simulink model "ep3_1"  (R2018a)
settings: Solver=VariableStepAuto  StartTime=0.0  StopTime=10.0  RelTol=1e-3
settings Model: Creator=zheny  LastModifiedBy=zheny

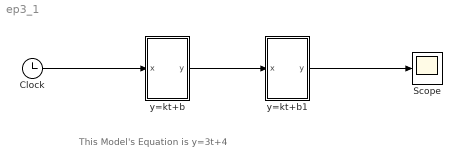
== system ep3_1 ==
  note: This Model's Equation is
      | y=3t+4
  Clock : Clock
  Scope : Scope
  y=kt+b : Subsystem  mask(y=kx+b){k=3, b=4}
      mask help: y=kx+b
      mask Help: y=kx+b
      mask Display: plot([0:0.1:1], [0:0.1:1]);
  y=kt+b1 : Subsystem  mask(y=kx+b){k=10, b=14}
      mask help: y=kx+b
      mask Help: y=kx+b
      mask Display: plot([0:0.1:1], [0:0.1:1]);
  wires:
  Clock/1 -> y=kt+b/1(x)
  y=kt+b/1(y) -> y=kt+b1/1(x)
  y=kt+b1/1(y) -> Scope/1

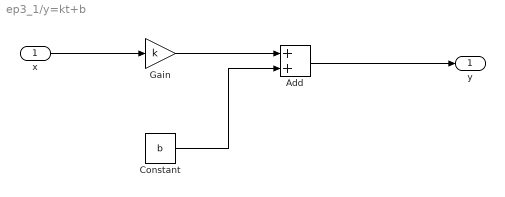
== system ep3_1/y=kt+b ==
  x : Inport
  Add : Sum
  Constant : Constant  Value=b
  Gain : Gain  Gain=k
  y : Outport
  wires:
  Constant/1 -> Add/2
  x/1 -> Gain/1
  Gain/1 -> Add/1
  Add/1 -> y/1

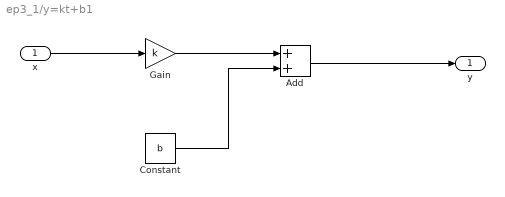
== system ep3_1/y=kt+b1 ==
  x : Inport
  Add : Sum
  Constant : Constant  Value=b
  Gain : Gain  Gain=k
  y : Outport
  wires:
  Constant/1 -> Add/2
  x/1 -> Gain/1
  Gain/1 -> Add/1
  Add/1 -> y/1
